simulink model "Ghost_f234"  (Simulink 8.1)
settings: Solver=ode1  StartTime=0.0  StopTime=inf  FixedStep=Ts  MaxStep=1e-3  RelTol=1e-3
PostLoadFcn:
  | NREL_Mode=1; BANSHEE_init;
InitFcn:
  | NREL_Mode=1; BANSHEE_init;
values from neighbouring files (symbols this model uses):
  DER_REL = xlsread('DER_relay.xlsx')    [relay_settings_init.m]
  F0 = xlsread('F0_relay_banshee.xlsx')    [relay_settings_init.m]
  F2 = xlsread('F2_relay_banshee.xlsx')    [relay_settings_init.m]
  F3 = xlsread('F3_relay_banshee.xlsx')    [relay_settings_init.m]
  F4 = xlsread('F4_relay_nrel.xlsx')    [relay_settings_init.m]
  Ts = 100E-6    (= 0.0001)    [BANSHEE_init.m]    (also in Ghost_init.m)
undefined symbols (not defined in the file or in its folder): CBID, communications_lib, Feeder2_lib, Feeder3_lib, Feeder4_lib, generic_ethernet_cb, Left, relay_housing_lib, SM_UtilityService, SS_COMMUNICATION, SS_F2_RELAY_HOUSING, SS_F3_RELAY_HOUSING, SS_Feeder2, SS_Feeder3, SS_Feeder4, Stim, type, utility_service_lib, V
libraries: simulink x80, relay_modbus_lib x80, breaker_lib x46, rtio_generic_modbus x45, cables_lib x30, rtlab x22, Load_lib x21, powerlib x20, transformer_lib x19, ssn_lib x13, artemis x6, BESS_lib x4
(part 1 of 6)
settings Model: ARTEMISmethode_block_infos=$$__separator__$$Ghost_f234/ARTEMIS Guide$$__separator__$$  Creator=RE25624  LastModifiedBy=hptb1  BufferReuse=off
settings SolverCC: ZeroCrossAlgorithm=Adaptive
settings DataIOCC: ExternalInput=getinputstruct(op_snapshot1)  InitialState=getstatestruct(op_snapshot1)  LimitDataPoints=off  MaxDataPoints=90060  SignalLoggingSaveFormat=Dataset  SaveOutput=off  SignalLogging=off  DSMLogging=off  SaveTime=off  OutputSaveName=result
settings OptimizationCC: BlockReduction=off  OptimizeBlockIOStorage=off  BufferReuse=off  ExpressionFolding=off  LocalBlockOutputs=off
settings DebuggingCC: MaxConsecutiveZCsMsg=warning  IgnoredZcDiagnostic=none  SolverPrmCheckMsg=none  MultiTaskRateTransMsg=warning  ParameterPrecisionLossMsg=none  FcnCallInpInsideContextMsg=EnableAllAsWarning  FrameProcessingCompatibilityMsg=error  ModelReferenceExtraNoncontSigs=warning  StrictBusMsg=Warning
settings ModelReferenceCC: UpdateModelReferenceTargets=IfOutOfDate
settings SFSimCC: SFSimEcho=off
settings GRTTargetCC: CodeReplacementLibrary=C89/C90 (ANSI)

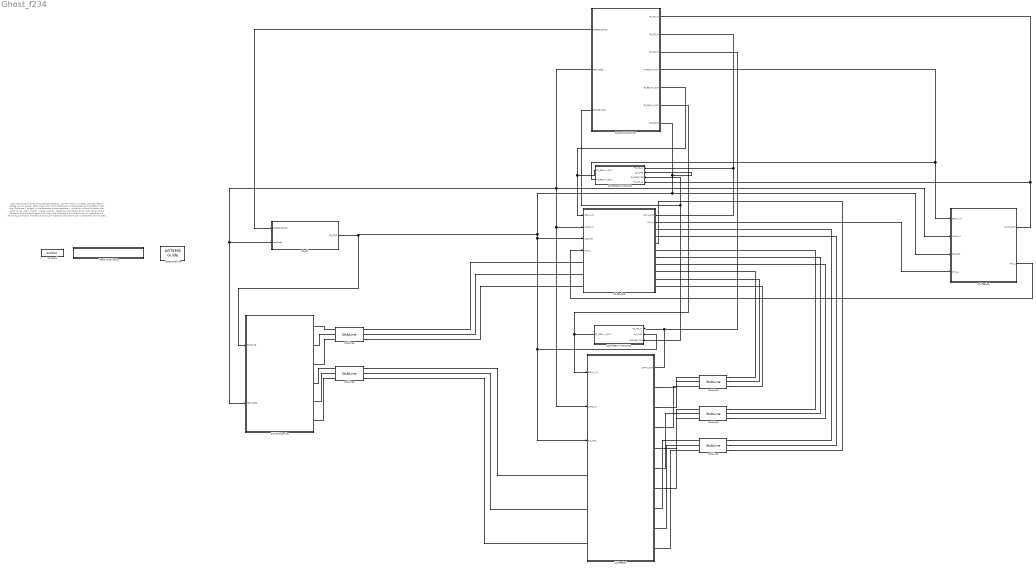
== system Ghost_f234 ==
  note: Copyright 2018 Alliance for Sustainable Energy, LLC
      |
      | Permission is hereby granted, free of charge, to any person obtaining a copy of this software
      | and associated documentation files (the "Software"), to deal in the Software without restriction,
      | including without limitation the rights to use, copy, modify, merge, publish, distribute, sublicense,
      | and/or sell copies of the Software, and to permit persons to whom the Software is furnished to do so,
      | subject to the following conditions:
      |
      | The above copyright notice and this permission notice shall be included in all copies or substantial portions of the Software.
      |
      | THE SOFTWARE IS PROVIDED "AS IS", WITHOUT WARRANTY OF ANY KIND, EXPRESS OR IMPLIED, INCLUDING
      | BUT NOT LIMITED TO THE WARRANTIES OF MERCHANTABILITY, FITNESS FOR A PARTICULAR PURPOSE AND
      | NONINFRINGEMENT. IN NO EVENT SHALL THE AUTHORS, THE COPYRIGHT HOLDERS, THE UNITED STATES,
      | THE UNITED STATES DEPARTMENT OF ENERGY, OR ANY OF THEIR EMPLOYEES BE LIABLE FOR ANY CLAIM,
      | DAMAGES OR OTHER LIABILITY, WHETHER IN AN ACTION OF CONTRACT, TORT OR OTHERWISE, ARISING FROM,
      | OUT OF OR IN CONNECTION WITH THE SOFTWARE OR THE USE OR OTHER DEALINGS IN THE SOFTWARE.
  ARTEMIS Guide : artemis/ARTEMIS/ARTEMIS Guide  Tag=FTSSmethode_opal_4hx0r99  Description=5.0_z1  lock=on  Ts=Ts  opt=art5  dyna=off  nb_perm=4  RT_fullcomp=off  ssn=on  ssn_itvc=off  ssn_ivic=off  ssn_ext=off  ssn_solver=Art5 with Backward Euler nodal interface  ssn_impulse=off  ssn_quasimpulse=off  ssn_impulse_loop=5  paraExtinctionThy=off  Thy_Impulse=on  dtc=Off  dtc_opt=normal  ao=on  simtype=off  ct_mac=off  lin_mov=off  lsp=[0.001 2]  spike_skip=Disabled  dtc_extra=1  dtc_sws=normal  dtc_pied=0.5  SPSRulesBlock=SPSRules  tre=on  ctmm=off  LF=off  dpl_type=ARTEMiS DPL  rlc_type=off  custom_type=off  para=on  ssn_ImpulseLoopBlockedStateUpdate=5  ssn_mov_iter_number=5  ssn_switch_iter_number=5  ssn_nib_type_verify=on
  Model Initialization : Subsystem  AncestorBlock=artemis/Tools /Misc/Model Initialization  mask(Model Functions){InitFcnX=NREL_Mode=1; BANSHEE_init;, prel=off, posl=on, inif=on, strf=off}
      mask prompts: InitFcnX "Initialisation"; prel "Preload Function"; posl "PostLoad Function"; inif "InitFcn"; strf "StartFcn"
      mask init:
      | currentBlock = gcb;
      | root = bdroot(currentBlock);
      | 
      | if ~strcmp(get_param(root,'BlockDiagramType'),'library')
      |     if prel==1
      |         set_param(root, 'PreLoadFcn', InitFcnX);
      |     else
      |         set_param(root, 'PreLoadFcn', '');
      |     end
      |     if inif==1
      |         set_param(root, 'InitFcn', InitFcnX);
      |     else
      |         set_param(root, 'InitFcn', '');
      |     end
      |     if strf==1
      |         set_param(root, 'StartFcn', InitFcnX);
      |     else
      |         set_param(root, 'StartFcn', '');
      |     end
      |     if posl==1
      |         set_param(root, 'PostLoadFcn', InitFcnX);
      |     else
      |         set_param(root, 'PostLoadFcn', '');
      |     end
      | end
      | 
      | pos = get_param(currentBlock, 'Position');
      | width = pos(3) - pos(1); height = pos(4) - pos(2);
      | txt = [ upper(root) '\n' '- InitFcn. . . . . '  get_param(root, 'InitFcn') ];
      settings: CopyFcn=set_param(gcb,'LinkStatus','inactive')
      mask Display: text(5, height*0.5, txt, 'horizontalAlignment', 'left', 'verticalAlignment', 'middle') ;
  SC_ctrl : Subsystem
  SM_UtilityService : Subsystem  AncestorBlock=utility_service_lib/SM_UtilityService
  SS_COMMUNICATION : Subsystem  AncestorBlock=communications_lib/SS_COMMUNICATION
  SS_F2_RELAY_HOUSING : Subsystem  AncestorBlock=relay_housing_lib/SS_F2_RELAY_HOUSING
  SS_F3_RELAY_HOUSING : Subsystem  AncestorBlock=relay_housing_lib/SS_F3_RELAY_HOUSING
  SS_Feeder2 : Subsystem  AncestorBlock=Feeder2_lib/SS_Feeder2
  SS_Feeder3 : Subsystem  AncestorBlock=Feeder3_lib/SS_Feeder3
  SS_Feeder4 : Subsystem  AncestorBlock=Feeder4_lib/SS_Feeder4
  StubLine1 : artemis/ARTEMIS/StubLine  Phases=3  pu=off  L=1500 * 9.43453e-08 / 2  Lpu=0.08  R=1500 * 2.28409e-5 / 2  Rpu=0.002  S_base=450e6/3  V_base=230e3/sqrt(3)  F_base=60  Ts=Ts
  StubLine2 : artemis/ARTEMIS/StubLine  Phases=3  pu=off  L=1500 * 9.43453e-08 / 2  Lpu=0.08  R=1500 * 2.28409e-5 / 2  Rpu=0.002  S_base=450e6/3  V_base=230e3/sqrt(3)  F_base=60  Ts=Ts
  StubLine3 : artemis/ARTEMIS/StubLine  Phases=3  pu=off  L=1500 * 9.43453e-08 / 2  Lpu=0.08  R=1500 * 2.28409e-5 / 2  Rpu=0.002  S_base=450e6/3  V_base=230e3/sqrt(3)  F_base=60  Ts=Ts
  StubLine8 : artemis/ARTEMIS/StubLine  Phases=3  pu=on  L=1500 * 9.43453e-08 / 2  Lpu=0.08  R=1500 * 2.28409e-5 / 2  Rpu=0.002  S_base=50e6/3  V_base=13.8e3/sqrt(3)  F_base=60  Ts=Ts
  StubLine9 : artemis/ARTEMIS/StubLine  Phases=3  pu=on  L=1500 * 9.43453e-08 / 2  Lpu=0.08  R=1500 * 2.28409e-5 / 2  Rpu=0.002  S_base=50e6/3  V_base=13.8e3/sqrt(3)  F_base=60  Ts=Ts
  powergui : powerlib/powergui  Priority=2  SimulationMode=Discrete  SolverType=Tustin  SampleTime=Ts  frequency=60  SPID=off  DisableSnubberDevices=off  DisableRonSwitches=off  DisableVfSwitches=off  SwTol=0  Interpol=off  DisplayEquations=off  frequencyindice=0  Pbase=100e6  ErrMax=1e-4  Iterations=50  UnitsV=kV  UnitsW=MW  FunctionMessages=off  echomessages=off  HookPort=off  EnableUseOfTLC=off  x0status=blocks  RestoreLinks=warning  ResistiveCurrentMeasurement=off  Frange=logspace(0,3,50)  Ylog=off  Xlog=off  ShowGrid=off  save=off  variable=ZData  structure=0  ZoomFFT=on  StartTime=0.0  cycles=2  DisplayStyle=off  fundamental=60  FreqAxis=off  MaxFrequency=1000  frequencyindicesteady=1  RmsSteady=1  display=off  Ts=0  methode=off
  wires:
  SS_Feeder3/1(DATA_OUT) -> SS_COMMUNICATION/2(F3_MS_IN), SS_F3_RELAY_HOUSING/1(F3_MS_IN)
  SS_F3_RELAY_HOUSING/1(F3_RELAY _OUT) -> SS_COMMUNICATION/5(F3_RELAY_OUT), SS_Feeder3/1(RELAY_IN)
  SS_F2_RELAY_HOUSING/1(F2_RELAY _OUT) -> SS_COMMUNICATION/6(F2_RELAY_OUT), SS_Feeder2/1(RELAY_IN)
  SS_Feeder2/1(DATA_OUT) -> SS_COMMUNICATION/3(F2_MS_IN), SS_F2_RELAY_HOUSING/1(F2_MS_IN)
  SS_COMMUNICATION/1(CMBNE_SGNLS) -> SC_ctrl/1(CMBNE_SGNLS)
  SC_ctrl/1(SC_CMD) -> SS_F2_RELAY_HOUSING/2(SC_CMD), SS_Feeder2/3(SC_CMD), SS_Feeder3/3(SC_CMD), SS_Feeder4/3(SC_CMD), SS_COMMUNICATION/7(CONSOLE), SS_F3_RELAY_HOUSING/2(SC_CMD), SM_UtilityService/1(CONSOLE)
  SS_F3_RELAY_HOUSING/2(F4_RELAY _OUT) -> SS_Feeder4/1(RELAY_IN), SS_COMMUNICATION/4(F4_RELAY_OUT)
  SS_Feeder4/1(DATA_OUT) -> SS_COMMUNICATION/1(F4_MS_IN), SS_F3_RELAY_HOUSING/4(F4_MS_IN)
  SS_Feeder3/2(PHIL_V) -> SS_Feeder4/4(PHIL_V)
  SS_Feeder4/2(PHIL_I) -> SS_Feeder3/4(PHIL_I)
  SS_COMMUNICATION/3(GOOSE_TRIP) -> SS_F3_RELAY_HOUSING/3(GOOSE_TRIP), SS_F2_RELAY_HOUSING/3(GOOSE_TRIP)
  SS_COMMUNICATION/2(TEST_SEQ) -> SS_Feeder2/2(LOAD_IN), SS_Feeder3/2(LOAD_IN), SM_UtilityService/2(TEST_SEQ), SC_ctrl/2(TestData), SS_Feeder4/2(LOAD_IN)
  connections:
  SS_Feeder2/RConn2 -- StubLine1/LConn2
  SS_Feeder2/RConn1 -- StubLine1/LConn1
  SS_Feeder2/RConn3 -- StubLine1/LConn3
  StubLine2/LConn2 -- SS_Feeder2/RConn5
  StubLine2/LConn3 -- SS_Feeder2/RConn6
  StubLine2/LConn1 -- SS_Feeder2/RConn4
  StubLine3/LConn2 -- SS_Feeder2/RConn8
  StubLine3/LConn1 -- SS_Feeder2/RConn7
  StubLine3/LConn3 -- SS_Feeder2/RConn9
  StubLine3/RConn3 -- SS_Feeder3/RConn3
  StubLine3/RConn2 -- SS_Feeder3/RConn2
  StubLine3/RConn1 -- SS_Feeder3/RConn1
  StubLine2/RConn3 -- SS_Feeder3/RConn6
  StubLine2/RConn1 -- SS_Feeder3/RConn4
  StubLine1/RConn3 -- SS_Feeder3/RConn9
  StubLine1/RConn2 -- SS_Feeder3/RConn8
  StubLine1/RConn1 -- SS_Feeder3/RConn7
  StubLine8/LConn1 -- SM_UtilityService/RConn1
  StubLine8/LConn2 -- SM_UtilityService/RConn2
  StubLine8/LConn3 -- SM_UtilityService/RConn3
  StubLine9/LConn2 -- SM_UtilityService/RConn5
  StubLine9/LConn3 -- SM_UtilityService/RConn6
  StubLine9/LConn1 -- SM_UtilityService/RConn4
  StubLine8/RConn3 -- SS_Feeder3/LConn3
  StubLine8/RConn2 -- SS_Feeder3/LConn2
  StubLine8/RConn1 -- SS_Feeder3/LConn1
  StubLine9/RConn1 -- SS_Feeder2/LConn1
  StubLine9/RConn2 -- SS_Feeder2/LConn2
  StubLine9/RConn3 -- SS_Feeder2/LConn3
  SS_Feeder3/RConn5 -- StubLine2/RConn2

== system Ghost_f234/Model Initialization ==

== system Ghost_f234/SC_ctrl ==
  note: % Copyright (c) 2016 Massachusetts Institute of Technology
      | % Permission is hereby granted, free of charge, to any person obtaining a copy of this
      | % software and associated documentation files (the "Software"), to deal in the Software
      | % without restriction, including without limitation the rights to use, copy, modify,
      | % merge, publish, distribute, sublicense, and/or sell copies of the Software, and to
      | % permit persons to whom the Software is furnished to do so, subject to the following
      | % conditions:
      | %
      | %
      | % The above copyright notice and this permission notice shall be included in
      | % all copies or substantial portions of the Software.
      | %
      | % THE SOFTWARE IS PROVIDED "AS IS", WITHOUT WARRANTY OF ANY KIND, EXPRESS OR IMPLIED,
      | % INCLUDING BUT NOT LIMITED TO THE WARRANTIES OF MERCHANTABILITY, FITNESS FOR A
      | % PARTICULAR PURPOSE AND NONINFRINGEMENT. IN NO EVENT SHALL THE AUTHORS OR COPYRIGHT
      | % HOLDERS BE LIABLE FOR ANY CLAIM, DAMAGES OR OTHER LIABILITY, WHETHER IN AN ACTION
      | % OF CONTRACT, TORT OR OTHERWISE, ARISING FROM, OUT OF OR IN CONNECTION WITH THE
      | % SOFTWARE OR THE USE OR OTHER DEALINGS IN THE SOFTWARE.
      | %
      | %
      | %%
  CMBNE_SGNLS : Inport
  TestData : Inport  Port=2
  Bus Creator1 : BusCreator  Inputs=11
  Bus Creator2 : BusCreator  Inputs=2
  Bus Selector : BusSelector  OutputSignals=F2_MS_IN
  Bus Selector{6..7,10,12,14} (5 alike) : BusSelector  OutputSignals=Status
  Bus Selector11 : BusSelector  OutputSignals=F3_MS_IN.CB_DATA.F3_PCC,F3_MS_IN.CB_DATA.F3_CB_10
  Bus Selector13 : BusSelector  OutputSignals=ESS_DATA
  Bus Selector15 : BusSelector  OutputSignals=Battery.SoC
  Bus Selector16 : BusSelector  OutputSignals=F4_MS_IN
  Bus Selector17 : BusSelector  OutputSignals=ESS_DATA
  Bus Selector18 : BusSelector  OutputSignals=Battery.SoC
  Bus Selector5 : BusSelector  OutputSignals=F3_MS_IN.CB_DATA.F3_PCC,F3_MS_IN.CB_DATA.F3_CB_3,F3_MS_IN.NG_CHP_DATA
  Bus Selector8 : BusSelector  OutputSignals=cb.cb_meas
  CB_modbus_mock : Subsystem
  DO NOT WRITE : Constant  Value=0
  Gen1_Modbus_Stimuli2 : Subsystem
  Gen2_NGCHP_Modbus_Stimuli : Subsystem
  Gen3_Modbus_Stimuli1 : Subsystem
  IO_scaling : Subsystem
  Logical Operator1 : Logic  Inputs=3  AllPortsSameDT=off  OutDataTypeStr=boolean
  Logical Operator2 : Logic  Inputs=3  AllPortsSameDT=off  OutDataTypeStr=boolean
  Manual Switch : ManualSwitch
  Manual Switch1 : ManualSwitch
  OpComm : rtlab/OpComm  nbport=2  groupe_acq=1  subsys_rate=0  st=0  Synchronization=on  Interpolation=on  Threshold=1.0  Missed_Data=off  Sim_Time=off  Samples=off  dynSigOut=off  from_console=0  warning_done=off  writeOpCommFile=off  Offset=off
  PV1 control : Subsystem
  PV2 control : Subsystem
  Plots : Subsystem
  SOC1 control : Subsystem
  SOC2 control : Subsystem
  TestSeq : Subsystem
  TestSequenceGen : Subsystem
  WRITE : Constant
  SC_CMD : Outport
  wires:
  CMBNE_SGNLS/1 -> OpComm/1
  Bus Creator1/1 -> SC_CMD/1
  Manual Switch/1 -> Bus Creator2/1  "record_rms_signals"
  Manual Switch1/1 -> Bus Creator2/2  "record_inst_signals"
  Bus Creator2/1 -> [data_logging]  "DataLogging"
  TestData/1 -> OpComm/2
  WRITE/1 -> Manual Switch1/2, Manual Switch/2  "record_rms_signals"
  DO NOT WRITE/1 -> Manual Switch1/1, Manual Switch/1
  [data_logging] -> Bus Creator1/4  "DataLogging"
  CB_modbus_mock/1(Out1) -> Bus Creator1/7  "CBStimuli"
  Gen1_Modbus_Stimuli2/1(MbCtrl) -> Bus Creator1/8  "Gen1"
  SOC2 control/1(Out1) -> Bus Creator1/5  "ESS2_ctrl"
  PV2 control/1(Out1) -> Bus Creator1/6  "PV2_ctrl"
  OpComm/1 -> [CMBNE], Bus Selector11/1, Bus Selector5/1, Plots/1(CMBNE_SGNLS)
  Gen2_NGCHP_Modbus_Stimuli/1(MbCtrl) -> Bus Creator1/9  "CHP_cmds"
  Bus Selector5/1 -> Bus Selector6/1  "<F3_PCC>"
  Bus Selector5/3 -> Bus Selector8/1  "<NG_CHP_DATA>"
  Bus Selector6/1 -> Logical Operator1/1  "<Status>"
  Bus Selector7/1 -> Logical Operator1/3  "<Status>"
  Bus Selector8/1 -> Bus Selector7/1  "<cb_meas>"
  Logical Operator1/1 -> Gen2_NGCHP_Modbus_Stimuli/1(MainsCon)
  Bus Selector10/1 -> Logical Operator1/2  "<Status>"
  Bus Selector5/2 -> Bus Selector10/1  "<F3_CB_3>"
  Gen3_Modbus_Stimuli1/1(MbCtrl) -> Bus Creator1/10  "Gen3_ctrl"
  Logical Operator2/1 -> Gen3_Modbus_Stimuli1/1(MainsCon)
  Bus Selector11/1 -> Bus Selector12/1  "<F3_PCC>"
  Bus Selector12/1 -> Logical Operator2/1  "<Status>"
  Bus Selector11/2 -> Bus Selector14/1  "<F3_CB_10>"
  Bus Selector14/1 -> Logical Operator2/3, Logical Operator2/2  "<Status>"
  OpComm/2 -> TestSeq/1(TestData)
  IO_scaling/1(Out1) -> Bus Creator1/11  "IO_scaling"
  TestSequenceGen/1(Out1) -> Bus Creator1/1  "TestSeq"
  SOC1 control/1(Out1) -> Bus Creator1/2  "ESS1_ctrl"
  PV1 control/1(Out1) -> Bus Creator1/3  "PV1_ctrl"
  [CMBNE] -> Bus Selector/1
  Bus Selector/1 -> Bus Selector13/1  "<F2_MS_IN>"
  Bus Selector13/1 -> Bus Selector15/1  "<ESS_DATA>"
  Bus Selector15/1 -> SOC1 control/1(SOC)  "<SoC>"
  [CMBNE] -> Bus Selector16/1
  Bus Selector16/1 -> Bus Selector17/1  "<F4_MS_IN>"
  Bus Selector17/1 -> Bus Selector18/1  "<ESS_DATA>"
  Bus Selector18/1 -> SOC2 control/1(SOC)  "<SoC>"

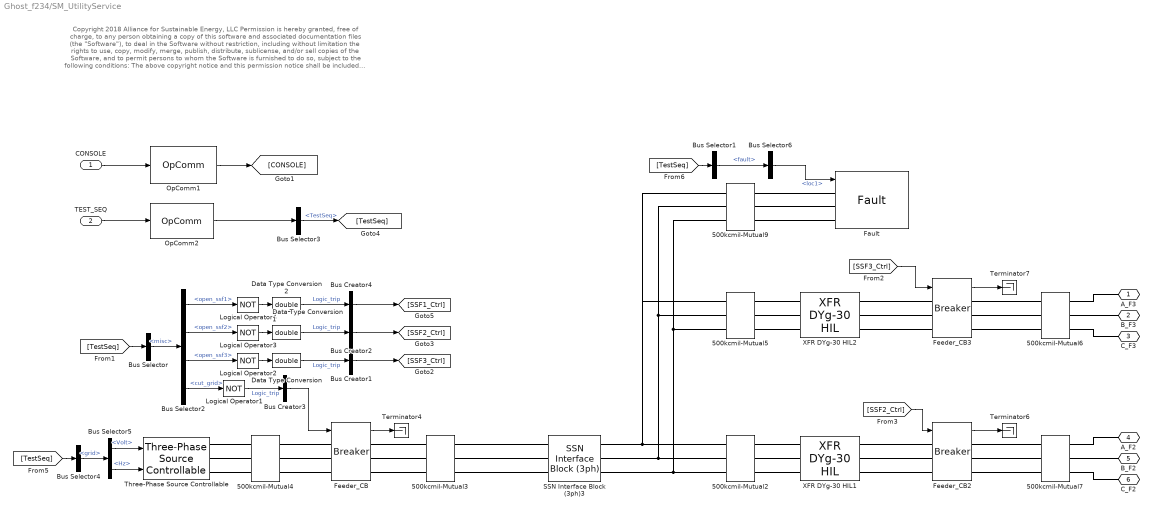
== system Ghost_f234/SM_UtilityService ==
  note: Copyright 2018 Alliance for Sustainable Energy, LLC
      |
      | Permission is hereby granted, free of charge, to any person obtaining a copy of this software
      | and associated documentation files (the "Software"), to deal in the Software without restriction,
      | including without limitation the rights to use, copy, modify, merge, publish, distribute, sublicense,
      | and/or sell copies of the Software, and to permit persons to whom the Software is furnished to do so,
      | subject to the following conditions:
      |
      | The above copyright notice and this permission notice shall be included in all copies or substantial portions of the Software.
      |
      | THE SOFTWARE IS PROVIDED "AS IS", WITHOUT WARRANTY OF ANY KIND, EXPRESS OR IMPLIED, INCLUDING
      | BUT NOT LIMITED TO THE WARRANTIES OF MERCHANTABILITY, FITNESS FOR A PARTICULAR PURPOSE AND
      | NONINFRINGEMENT. IN NO EVENT SHALL THE AUTHORS, THE COPYRIGHT HOLDERS, THE UNITED STATES,
      | THE UNITED STATES DEPARTMENT OF ENERGY, OR ANY OF THEIR EMPLOYEES BE LIABLE FOR ANY CLAIM,
      | DAMAGES OR OTHER LIABILITY, WHETHER IN AN ACTION OF CONTRACT, TORT OR OTHERWISE, ARISING FROM,
      | OUT OF OR IN CONNECTION WITH THE SOFTWARE OR THE USE OR OTHER DEALINGS IN THE SOFTWARE.
  CONSOLE : Inport
  TEST_SEQ : Inport  Port=2
  500kcmil-Mutual2 : cables_lib/500kcmil-Mutual  length=200  par_sets=1  ratio=3
  500kcmil-Mutual{3..4,6..7} (4 alike) : cables_lib/500kcmil-Mutual  length=50  par_sets=1  ratio=3
  500kcmil-Mutual5 : cables_lib/500kcmil-Mutual  length=200  par_sets=1  ratio=3
  500kcmil-Mutual9 : cables_lib/500kcmil-Mutual  length=200  par_sets=1  ratio=3
  Bus Creator{1..4} (4 alike) : BusCreator  Inputs=1
  Bus Selector : BusSelector  OutputSignals=misc
  Bus Selector1 : BusSelector  OutputSignals=fault
  Bus Selector2 : BusSelector  OutputSignals=open_ssf1,open_ssf2,open_ssf3,cut_grid
  Bus Selector3 : BusSelector  OutputSignals=TestSeq
  Bus Selector4 : BusSelector  OutputSignals=grid
  Bus Selector5 : BusSelector  OutputSignals=Volt,Hz
  Bus Selector6 : BusSelector  OutputSignals=loc1
  Data Type Conversion : DataTypeConversion  OutDataTypeStr=double
  Data Type Conversion1 : DataTypeConversion  OutDataTypeStr=double
  Data Type Conversion2 : DataTypeConversion  OutDataTypeStr=double
  Fault : fault_lib/Fault  FaultResistance=0.1  GroundResistance=1.73  SnubberResistance=1E6
  Feeder_CB : breaker_lib/Breaker  Ts=Ts  mech_delay=cb_mech_delay
  Feeder_CB2 : breaker_lib/Breaker  Ts=Ts  mech_delay=cb_mech_delay
  Feeder_CB3 : breaker_lib/Breaker  Ts=Ts  mech_delay=cb_mech_delay
  Logical Operator{1..4} (4 alike) : Logic  Operator=NOT  AllPortsSameDT=off  OutDataTypeStr=boolean
  OpComm1 : rtlab/OpComm  nbport=1  groupe_acq=1  subsys_rate=0  st=0  Synchronization=on  Interpolation=on  Threshold=1.0  Missed_Data=off  Sim_Time=off  Samples=off  dynSigOut=off  from_console=1  warning_done=off  writeOpCommFile=off  Offset=off
  OpComm2 : rtlab/OpComm  nbport=1  groupe_acq=1  subsys_rate=0  st=0  Synchronization=on  Interpolation=on  Threshold=1.0  Missed_Data=off  Sim_Time=off  Samples=off  dynSigOut=off  from_console=0  warning_done=off  writeOpCommFile=off  Offset=off
  SSN Interface Block (3ph)3 : ssn_lib/SSN Interface Block (3ph)  nb_phase=3  nb_port=2  p1_type=V-type(Left)  p2_type=V-type (Right)  p3_type=V-type(Left)  p4_type=V-type(Left)  p5_type=V-type(Left)  p6_type=V-type(Left)  p7_type=V-type(Left)  p8_type=V-type(Left)  p9_type=V-type(Left)  p10_type=V-type(Left)  p11_type=V-type(Left)  p12_type=V-type(Left)  p13_type=V-type(Left)  p14_type=V-type(Left)  p15_type=V-type(Left)  p16_type=V-type(Left)  I_port_shunt_resistance=1e9
  Terminator4 : Terminator
  Terminator6 : Terminator
  Terminator7 : Terminator
  Three-Phase Source Controllable : controllable_grid_lib/Three-Phase Source Controllable  Ts=Ts  Rg=0.8  Lg=16.58e-3  mask{Ts=Ts}
  XFR DYg-30 HIL1 : transformer_lib/XFR DYg-30 HIL  Rating=50000  Vp=115000  Vs=13800  Z=6  XR=30
  XFR DYg-30 HIL2 : transformer_lib/XFR DYg-30 HIL  Rating=50000  Vp=115000  Vs=13800  Z=6  XR=30
  A_F3 : PMIOPort  Port=1  Side=Right
  B_F3 : PMIOPort  Port=2  Side=Right
  C_F3 : PMIOPort  Port=3  Side=Right
  A_F2 : PMIOPort  Port=4  Side=Right
  B_F2 : PMIOPort  Port=5  Side=Right
  C_F2 : PMIOPort  Port=6  Side=Right
  wires:
  CONSOLE/1 -> OpComm1/1
  OpComm1/1 -> [CONSOLE]
  Feeder_CB/1 -> Terminator4/1
  Feeder_CB2/1 -> Terminator6/1
  Feeder_CB3/1 -> Terminator7/1
  TEST_SEQ/1 -> OpComm2/1
  [TestSeq] -> Bus Selector/1
  Logical Operator1/1 -> Bus Creator3/1  "Logic_trip"
  Bus Creator3/1 -> Feeder_CB/1
  Bus Selector/1 -> Bus Selector2/1  "<misc>"
  Bus Selector2/4 -> Logical Operator1/1  "<cut_grid>"
  Bus Selector2/3 -> Logical Operator2/1  "<open_ssf3>"
  Logical Operator2/1 -> Data Type Conversion/1
  Bus Creator1/1 -> [SSF3_Ctrl]
  Data Type Conversion/1 -> Bus Creator1/1  "Logic_trip"
  Bus Selector3/1 -> [TestSeq]  "<TestSeq>"
  OpComm2/1 -> Bus Selector3/1
  Bus Selector2/2 -> Logical Operator3/1  "<open_ssf2>"
  Logical Operator3/1 -> Data Type Conversion1/1
  Bus Creator2/1 -> [SSF2_Ctrl]
  Data Type Conversion1/1 -> Bus Creator2/1  "Logic_trip"
  Bus Selector2/1 -> Logical Operator4/1  "<open_ssf1>"
  Logical Operator4/1 -> Data Type Conversion2/1
  Bus Creator4/1 -> [SSF1_Ctrl]
  Data Type Conversion2/1 -> Bus Creator4/1  "Logic_trip"
  [SSF3_Ctrl] -> Feeder_CB3/1
  [SSF2_Ctrl] -> Feeder_CB2/1
  [TestSeq] -> Bus Selector4/1
  Bus Selector4/1 -> Bus Selector5/1  "<grid>"
  Bus Selector5/2 -> Three-Phase Source Controllable/2  "<Hz>"
  Bus Selector5/1 -> Three-Phase Source Controllable/1  "<Volt>"
  [TestSeq] -> Bus Selector1/1
  Bus Selector1/1 -> Bus Selector6/1  "<fault>"
  Bus Selector6/1 -> Fault/1  "<loc1>"
  connections:
  500kcmil-Mutual3/LConn3 -- Feeder_CB/RConn3
  500kcmil-Mutual3/LConn1 -- Feeder_CB/RConn1
  500kcmil-Mutual3/LConn2 -- Feeder_CB/RConn2
  SSN Interface Block (3ph)3/LConn2 -- 500kcmil-Mutual3/RConn2
  SSN Interface Block (3ph)3/LConn1 -- 500kcmil-Mutual3/RConn1
  SSN Interface Block (3ph)3/LConn3 -- 500kcmil-Mutual3/RConn3
  500kcmil-Mutual4/RConn3 -- Feeder_CB/LConn3
  500kcmil-Mutual4/RConn2 -- Feeder_CB/LConn2
  500kcmil-Mutual4/RConn1 -- Feeder_CB/LConn1
  Three-Phase Source Controllable/RConn3 -- 500kcmil-Mutual4/LConn3
  Three-Phase Source Controllable/RConn1 -- 500kcmil-Mutual4/LConn1
  Three-Phase Source Controllable/RConn2 -- 500kcmil-Mutual4/LConn2
  500kcmil-Mutual2/RConn2 -- XFR DYg-30 HIL1/LConn2
  500kcmil-Mutual2/RConn1 -- XFR DYg-30 HIL1/LConn1
  500kcmil-Mutual2/RConn3 -- XFR DYg-30 HIL1/LConn3
  500kcmil-Mutual5/RConn2 -- XFR DYg-30 HIL2/LConn2
  500kcmil-Mutual5/RConn1 -- XFR DYg-30 HIL2/LConn1
  500kcmil-Mutual5/RConn3 -- XFR DYg-30 HIL2/LConn3
  SSN Interface Block (3ph)3/RConn1 -- 500kcmil-Mutual2/LConn1 -- 500kcmil-Mutual5/LConn1 -- 500kcmil-Mutual9/LConn1
  500kcmil-Mutual5/LConn2 -- SSN Interface Block (3ph)3/RConn2 -- 500kcmil-Mutual2/LConn2 -- 500kcmil-Mutual9/LConn2
  500kcmil-Mutual5/LConn3 -- SSN Interface Block (3ph)3/RConn3 -- 500kcmil-Mutual2/LConn3 -- 500kcmil-Mutual9/LConn3
  XFR DYg-30 HIL2/RConn1 -- Feeder_CB3/LConn1
  XFR DYg-30 HIL2/RConn2 -- Feeder_CB3/LConn2
  XFR DYg-30 HIL2/RConn3 -- Feeder_CB3/LConn3
  XFR DYg-30 HIL1/RConn3 -- Feeder_CB2/LConn3
  XFR DYg-30 HIL1/RConn2 -- Feeder_CB2/LConn2
  XFR DYg-30 HIL1/RConn1 -- Feeder_CB2/LConn1
  500kcmil-Mutual6/LConn2 -- Feeder_CB3/RConn2
  500kcmil-Mutual6/LConn3 -- Feeder_CB3/RConn3
  500kcmil-Mutual6/LConn1 -- Feeder_CB3/RConn1
  500kcmil-Mutual7/LConn2 -- Feeder_CB2/RConn2
  500kcmil-Mutual7/LConn3 -- Feeder_CB2/RConn3
  500kcmil-Mutual7/LConn1 -- Feeder_CB2/RConn1
  B_F2/RConn1 -- 500kcmil-Mutual7/RConn2
  A_F2/RConn1 -- 500kcmil-Mutual7/RConn1
  C_F2/RConn1 -- 500kcmil-Mutual7/RConn3
  B_F3/RConn1 -- 500kcmil-Mutual6/RConn2
  A_F3/RConn1 -- 500kcmil-Mutual6/RConn1
  C_F3/RConn1 -- 500kcmil-Mutual6/RConn3
  500kcmil-Mutual9/RConn2 -- Fault/LConn2
  500kcmil-Mutual9/RConn3 -- Fault/LConn3
  500kcmil-Mutual9/RConn1 -- Fault/LConn1

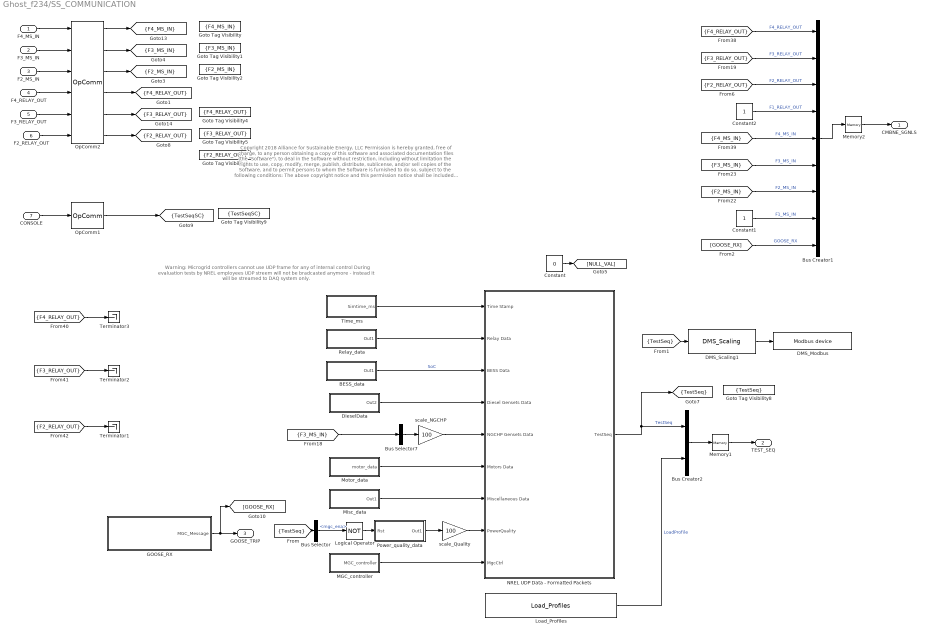
== system Ghost_f234/SS_COMMUNICATION ==
  note: Warning: Microgrid controllers cannot use UDP frame for any of internal control
      | During evaluation tests by NREL employees UDP streem will not be bradcasted anymore - instead it will
      | be streamed to DAQ system only.
  note: Copyright 2018 Alliance for Sustainable Energy, LLC
      |
      | Permission is hereby granted, free of charge, to any person obtaining a copy of this software
      | and associated documentation files (the "Software"), to deal in the Software without restriction,
      | including without limitation the rights to use, copy, modify, merge, publish, distribute, sublicense,
      | and/or sell copies of the Software, and to permit persons to whom the Software is furnished to do so,
      | subject to the following conditions:
      |
      | The above copyright notice and this permission notice shall be included in all copies or substantial portions of the Software.
      |
      | THE SOFTWARE IS PROVIDED "AS IS", WITHOUT WARRANTY OF ANY KIND, EXPRESS OR IMPLIED, INCLUDING
      | BUT NOT LIMITED TO THE WARRANTIES OF MERCHANTABILITY, FITNESS FOR A PARTICULAR PURPOSE AND
      | NONINFRINGEMENT. IN NO EVENT SHALL THE AUTHORS, THE COPYRIGHT HOLDERS, THE UNITED STATES,
      | THE UNITED STATES DEPARTMENT OF ENERGY, OR ANY OF THEIR EMPLOYEES BE LIABLE FOR ANY CLAIM,
      | DAMAGES OR OTHER LIABILITY, WHETHER IN AN ACTION OF CONTRACT, TORT OR OTHERWISE, ARISING FROM,
      | OUT OF OR IN CONNECTION WITH THE SOFTWARE OR THE USE OR OTHER DEALINGS IN THE SOFTWARE.
  F4_MS_IN : Inport
  F3_MS_IN : Inport  Port=2
  F2_MS_IN : Inport  Port=3
  F4_RELAY_OUT : Inport  Port=4
  F3_RELAY_OUT : Inport  Port=5
  F2_RELAY_OUT : Inport  Port=6
  CONSOLE : Inport  Port=7
  BESS_data : Subsystem
  Bus Creator1 : BusCreator  Inputs=9
  Bus Creator2 : BusCreator  Inputs=2
  Bus Selector : BusSelector  OutputSignals=misc.mgc_ena
  Bus Selector7 : BusSelector  OutputSignals=NG_CHP_DATA.cb.relay_out.m.Vpu,NG_CHP_DATA.CHPData.TempActual,NG_CHP_DATA.CHPData.Thermal data.Heat_Recovered_MBtu_hr,NG_CHP_DATA.CHPData.Thermal data.Nm3_per_hour_NG_fuel_usage,NG_CHP_DATA.CHPData.Thermal data.CO2_lbm_hr,NG_CHP_DATA.CHPData.HeatFromBoiler MBtu/hr,NG_CHP_DATA.CHPData.CHPHeatContribution MBtu/hr,NG_CHP_DATA.CHPData.Boiler_Nm^3/hr ,NG_CHP_DATA.CHPData.Boiler lbm/hr CO2  OutputAsBus=on
  Constant : Constant  Value=0
  Constant1 : Constant
  Constant2 : Constant
  DMS_Modbus : rtio_generic_modbus/Modbus device  conf_name=DMS_cfg.opal  conf_name_mask=DMS_cfg.xls  sample_time=Ts
  DMS_Scaling1 : DMS_slave_lib/DMS_Scaling
  DieselData : Subsystem
  "GOOSE_RX " : Subsystem
  Goto Tag Visibility : GotoTagVisibility  GotoTag=F4_MS_IN
  Goto Tag Visibility1 : GotoTagVisibility  GotoTag=F3_MS_IN
  Goto Tag Visibility2 : GotoTagVisibility  GotoTag=F2_MS_IN
  Goto Tag Visibility4 : GotoTagVisibility  GotoTag=F4_RELAY_OUT
  Goto Tag Visibility5 : GotoTagVisibility  GotoTag=F3_RELAY_OUT
  Goto Tag Visibility6 : GotoTagVisibility  GotoTag=F2_RELAY_OUT
  Goto Tag Visibility8 : GotoTagVisibility  GotoTag=TestSeq
  Goto Tag Visibility9 : GotoTagVisibility  GotoTag=TestSeqSC
  Load_Profiles : LoadProfiles_lib/Load_Profiles
  Logical Operator : Logic  Operator=NOT  AllPortsSameDT=off  OutDataTypeStr=boolean
  MGC_controller : Subsystem
  Memory1 : Memory
  Memory2 : Memory
  Misc_data : Subsystem
  Motor_data : Subsystem
  NREL UDP Data - Formatted Packets : Subsystem  AncestorBlock=NREL_UDP_lib/NREL UDP Data - Formatted Packets  mask(UDP Data Block){ProfileID=6, NumOfRelays=[59, [1, 1, 1000, 100]], NumOfBatteries=2, NumOfDieselGensets=[2, [100, 100]], NumOfNGCHPGensets=[1, [100, 100, 100, 100, 100, 100, 100, 100, 100]], NumOfMotors=2, NumOfQuality=[23 10 10], NumOfMiscellaneousDataScales=2, NumOfMiscellaneousDataSignalsScales=[[50, 1], [8, 1]]}
      mask prompts: ProfileID "Profile ID"; NumOfRelays "Relay Data"; NumOfBatteries "# of Batteries"; NumOfDieselGensets "Diesel Gensets Data"; NumOfNGCHPGensets "NG-CHP Gensets Data"; NumOfMotors "# of Motors"; NumOfQuality "Power quality"; NumOfMiscellaneousDataScales "Misc. Data - No. of Scale Factors"; NumOfMiscellaneousDataSignalsScales "Misc. - No. Signals and Scale Values"
      mask help:
      | * All signal scaling/modifications should be external to this block
      |
      | Profile ID: (1-Sheriff, 2-Banshee, 3-Canary, 4-Siren, 5-NREL)
      |
      | Relay Data: No. of relays feeding packet data to breakers in display - mapped/indexed in ascending order
      | -Packet order: Active power(kW), reactive power(kVAR), voltage(per-unit), frequency (Hz), breaker status (1:closed, 0:open)
      | -Input format: [No. of Relays, [scale_kW, scale_kVAR, scale_Vpu, scale_Hz]]
      | -Ex:[4, [10, 10, 100, 100]]
      |
      | No. of Batteries: TBD
      | -Ex: [0]
      |
      | No. of Diesel Gensets: No. of diesel gensets in the system feeding data to the display.
      | -Packet order: terminal voltage(per-unit), fuel consumption (Gals/hr)
      | -Input format: [No. of gensets, [scale_Vpu, scale_fuel]]
      | -Ex: [0, [1,1]]
      |
      | No. of NG/CHP Gensets: No. of NGCHP gensets in the system feeding data to the display.
      | -Packet order: Terminal Vpu, Temp Actual, Heat Recovered, Fuel usage, CHP CO2, Heat from boiler, CHP heat contribution, Boiler Nm^3/hr, Boiler lbm/hr CO2
      | -Ex: [1, [100,100,100,100,100,100,100,100,100]]
      |
      | Motors Data: No. of motors monitored in the system. Currently, only looking at motor on/off state.
      | -Input format: [No. of motors]
      | -Ex: [1]
      |
      | Misc. Data - No. of Scale factor: No. of scale factors to be applied to each signal-set.
      | -Ex: [3]
      |
      | Misc. Data - No. of Signals and Scale Values: Size of signal set and scale value to be applied to the signal-set.
      | -Ex: [[1, 1000], [6, 100], [3, 10]]
  OpComm1 : rtlab/OpComm  nbport=1  groupe_acq=1  subsys_rate=0  st=0  Synchronization=on  Interpolation=on  Threshold=1.0  Missed_Data=off  Sim_Time=off  Samples=off  dynSigOut=off  from_console=1  warning_done=off  writeOpCommFile=off  Offset=off
  OpComm2 : rtlab/OpComm  nbport=6  groupe_acq=1  subsys_rate=0  st=0  Synchronization=on  Interpolation=on  Threshold=1.0  Missed_Data=off  Sim_Time=off  Samples=off  dynSigOut=off  from_console=0  warning_done=off  writeOpCommFile=off  Offset=off
  Power_quality_data : Subsystem
  Relay_data : Subsystem
  Terminator1 : Terminator
  Terminator2 : Terminator
  Terminator3 : Terminator
  Time_ms : Subsystem
  scale_NGCHP : Gain  Gain=100
  scale_Quality : Gain  Gain=100
  CMBNE_SGNLS : Outport
  TEST_SEQ : Outport  Port=2
  GOOSE_TRIP : Outport  Port=3
  tag scope: F2_MS_IN=scoped, F2_RELAY_OUT=scoped, F3_MS_IN=scoped, F3_RELAY_OUT=scoped, F4_MS_IN=scoped, F4_RELAY_OUT=scoped, TestSeq=scoped, TestSeqSC=scoped
  wires:
  Load_Profiles/1 -> Bus Creator2/2  "LoadProfile"
  F3_MS_IN/1 -> OpComm2/2
  Memory1/1 -> TEST_SEQ/1
  F2_RELAY_OUT/1 -> OpComm2/6
  F2_MS_IN/1 -> OpComm2/3
  Constant/1 -> [NULL_VAL]
  [F3_MS_IN] -> Bus Selector7/1
  Bus Selector7/1 -> scale_NGCHP/1
  scale_NGCHP/1 -> NREL UDP Data - Formatted Packets/5(NGCHP Gensets Data)
  Memory2/1 -> CMBNE_SGNLS/1
  Bus Creator1/1 -> Memory2/1
  Constant1/1 -> Bus Creator1/8  "F1_MS_IN"
  [F2_RELAY_OUT] -> Bus Creator1/3  "F2_RELAY_OUT"
  Constant2/1 -> Bus Creator1/4  "F1_RELAY_OUT"
  [F3_RELAY_OUT] -> Bus Creator1/2  "F3_RELAY_OUT"
  [F3_MS_IN] -> Bus Creator1/6  "F3_MS_IN"
  [F2_MS_IN] -> Bus Creator1/7  "F2_MS_IN"
  Time_ms/1(Simtime_ms) -> NREL UDP Data - Formatted Packets/1(Time Stamp)
  F4_MS_IN/1 -> OpComm2/1
  F4_RELAY_OUT/1 -> OpComm2/4
  F3_RELAY_OUT/1 -> OpComm2/5
  OpComm2/1 -> [F4_MS_IN]
  OpComm2/2 -> [F3_MS_IN]
  OpComm2/3 -> [F2_MS_IN]
  OpComm2/4 -> [F4_RELAY_OUT]
  OpComm2/5 -> [F3_RELAY_OUT]
  OpComm2/6 -> [F2_RELAY_OUT]
  [F4_RELAY_OUT] -> Bus Creator1/1  "F4_RELAY_OUT"
  [F4_MS_IN] -> Bus Creator1/5  "F4_MS_IN"
  [F4_RELAY_OUT] -> Terminator3/1
  [F3_RELAY_OUT] -> Terminator2/1
  [F2_RELAY_OUT] -> Terminator1/1
  "GOOSE_RX "/1(MGC_Message) -> [GOOSE_RX], GOOSE_TRIP/1
  Relay_data/1(Out1) -> NREL UDP Data - Formatted Packets/2(Relay Data)
  Misc_data/1(Out1) -> NREL UDP Data - Formatted Packets/7(Miscellaneous Data)
  Motor_data/1(motor_data) -> NREL UDP Data - Formatted Packets/6(Motors Data)
  NREL UDP Data - Formatted Packets/1(TestSeq) -> [TestSeq], Bus Creator2/1  "TestSeq"
  Bus Creator2/1 -> Memory1/1
  CONSOLE/1 -> OpComm1/1
  OpComm1/1 -> [TestSeqSC]
  BESS_data/1(Out1) -> NREL UDP Data - Formatted Packets/3(BESS Data)  "SoC"
  DieselData/1(Out2) -> NREL UDP Data - Formatted Packets/4(Diesel Gensets Data)
  Power_quality_data/1(Out1) -> scale_Quality/1
  [TestSeq] -> Bus Selector/1
  Bus Selector/1 -> Logical Operator/1  "<mgc_ena>"
  Logical Operator/1 -> Power_quality_data/1(Rst)
  scale_Quality/1 -> NREL UDP Data - Formatted Packets/8("PowerQuality ")
  [TestSeq] -> DMS_Scaling1/1
  DMS_Scaling1/1 -> DMS_Modbus/1
  MGC_controller/1(MGC_controller) -> NREL UDP Data - Formatted Packets/9(MgcCtrl)
  [GOOSE_RX] -> Bus Creator1/9  "GOOSE_RX"

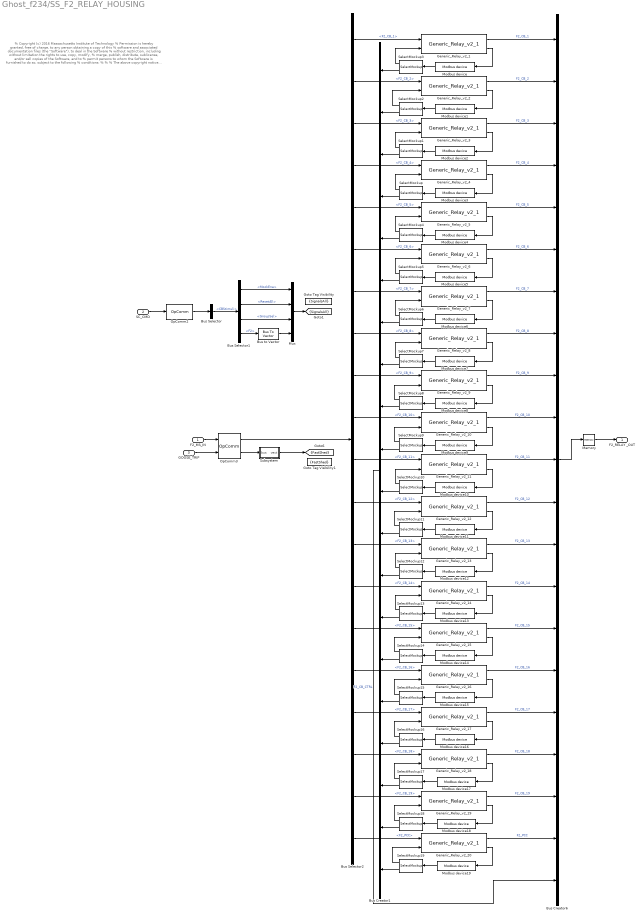
== system Ghost_f234/SS_F2_RELAY_HOUSING ==
  note: % Copyright (c) 2016 Massachusetts Institute of Technology
      | % Permission is hereby granted, free of charge, to any person obtaining a copy of this
      | % software and associated documentation files (the "Software"), to deal in the Software
      | % without restriction, including without limitation the rights to use, copy, modify,
      | % merge, publish, distribute, sublicense, and/or sell copies of the Software, and to
      | % permit persons to whom the Software is furnished to do so, subject to the following
      | % conditions:
      | %
      | %
      | % The above copyright notice and this permission notice shall be included in
      | % all copies or substantial portions of the Software.
      | %
      | % THE SOFTWARE IS PROVIDED "AS IS", WITHOUT WARRANTY OF ANY KIND, EXPRESS OR IMPLIED,
      | % INCLUDING BUT NOT LIMITED TO THE WARRANTIES OF MERCHANTABILITY, FITNESS FOR A
      | % PARTICULAR PURPOSE AND NONINFRINGEMENT. IN NO EVENT SHALL THE AUTHORS OR COPYRIGHT
      | % HOLDERS BE LIABLE FOR ANY CLAIM, DAMAGES OR OTHER LIABILITY, WHETHER IN AN ACTION
      | % OF CONTRACT, TORT OR OTHERWISE, ARISING FROM, OUT OF OR IN CONNECTION WITH THE
      | % SOFTWARE OR THE USE OR OTHER DEALINGS IN THE SOFTWARE.
      | %
      | %
      | %%
  F2_MS_IN : Inport
  SC_CMD : Inport  Port=2
  GOOSE_TRIP : Inport  Port=3
  Bus Creator1 : BusCreator  Inputs=20
  Bus Creator6 : BusCreator  Inputs=21
  Bus Selector : BusSelector  OutputSignals=CBStimuli
  Bus Selector1 : BusSelector  OutputSignals=MockEna,ResetAll,GroupSel,F2
  Bus Selector2 : BusSelector  OutputSignals=CB_DATA.F2_CB_1,CB_DATA.F2_CB_2,CB_DATA.F2_CB_3,CB_DATA.F2_CB_4,CB_DATA.F2_CB_5,CB_DATA.F2_CB_6,CB_DATA.F2_CB_7,CB_DATA.F2_CB_8,CB_DATA.F2_CB_9,CB_DATA.F2_CB_10,CB_DATA.F2_CB_11,CB_DATA.F2_CB_12,CB_DATA.F2_CB_13,CB_DATA.F2_CB_14,CB_DATA.F2_CB_15,CB_DATA.F2_CB_16,CB_DATA.F2_CB_17,CB_DATA.F2_CB_18,CB_DATA.F2_CB_19,CB_DATA.F2_PCC
  Bus to Vector : BusToVector
  Generic_Relay_v2_1 : relay_modbus_lib/Generic_Relay_v2_1  Ts=Ts  relay_settings=[F2(1,:)]
  Generic_Relay_v2_10 : relay_modbus_lib/Generic_Relay_v2_1  Ts=Ts  relay_settings=[F2(10,:)]
  Generic_Relay_v2_11 : relay_modbus_lib/Generic_Relay_v2_1  Ts=Ts  relay_settings=[F2(11,:)]
  Generic_Relay_v2_12 : relay_modbus_lib/Generic_Relay_v2_1  Ts=Ts  relay_settings=[F2(12,:)]
  Generic_Relay_v2_13 : relay_modbus_lib/Generic_Relay_v2_1  Ts=Ts  relay_settings=[F2(13,:)]
  Generic_Relay_v2_14 : relay_modbus_lib/Generic_Relay_v2_1  Ts=Ts  relay_settings=[F2(14,:)]
  Generic_Relay_v2_15 : relay_modbus_lib/Generic_Relay_v2_1  Ts=Ts  relay_settings=[F2(15,:)]
  Generic_Relay_v2_16 : relay_modbus_lib/Generic_Relay_v2_1  Ts=Ts  relay_settings=[F2(16,:)]
  Generic_Relay_v2_17 : relay_modbus_lib/Generic_Relay_v2_1  Ts=Ts  relay_settings=[F2(17,:)]
  Generic_Relay_v2_18 : relay_modbus_lib/Generic_Relay_v2_1  Ts=Ts  relay_settings=[F2(18,:)]
  Generic_Relay_v2_19 : relay_modbus_lib/Generic_Relay_v2_1  Ts=Ts  relay_settings=[F2(19,:)]
  Generic_Relay_v2_2 : relay_modbus_lib/Generic_Relay_v2_1  Ts=Ts  relay_settings=[F2(2,:)]
  Generic_Relay_v2_20 : relay_modbus_lib/Generic_Relay_v2_1  Ts=Ts  relay_settings=[F0(2,:)]
  Generic_Relay_v2_3 : relay_modbus_lib/Generic_Relay_v2_1  Ts=Ts  relay_settings=[F2(3,:)]
  Generic_Relay_v2_4 : relay_modbus_lib/Generic_Relay_v2_1  Ts=Ts  relay_settings=[F2(4,:)]
  Generic_Relay_v2_5 : relay_modbus_lib/Generic_Relay_v2_1  Ts=Ts  relay_settings=[F2(5,:)]
  Generic_Relay_v2_6 : relay_modbus_lib/Generic_Relay_v2_1  Ts=Ts  relay_settings=[F2(6,:)]
  Generic_Relay_v2_7 : relay_modbus_lib/Generic_Relay_v2_1  Ts=Ts  relay_settings=[F2(7,:)]
  Generic_Relay_v2_8 : relay_modbus_lib/Generic_Relay_v2_1  Ts=Ts  relay_settings=[F2(8,:)]
  Generic_Relay_v2_9 : relay_modbus_lib/Generic_Relay_v2_1  Ts=Ts  relay_settings=[F2(9,:)]
  Goto Tag Visibility : GotoTagVisibility  GotoTag=SignalsAll
  Goto Tag Visibility1 : GotoTagVisibility  GotoTag=FastShed
  Memory : Memory
  Modbus device : rtio_generic_modbus/Modbus device  conf_name=F2_relay_cfg1.opal  conf_name_mask=F2_relay_cfg1.xls  sample_time=Ts
  Modbus device1 : rtio_generic_modbus/Modbus device  conf_name=F2_relay_cfg2.opal  conf_name_mask=F2_relay_cfg2.xls  sample_time=Ts
  Modbus device10 : rtio_generic_modbus/Modbus device  conf_name=F2_relay_cfg11.opal  conf_name_mask=F2_relay_cfg11.xls  sample_time=Ts
  Modbus device11 : rtio_generic_modbus/Modbus device  conf_name=F2_relay_cfg12.opal  conf_name_mask=F2_relay_cfg12.xls  sample_time=Ts
  Modbus device12 : rtio_generic_modbus/Modbus device  conf_name=F2_relay_cfg13.opal  conf_name_mask=F2_relay_cfg13.xls  sample_time=Ts
  Modbus device13 : rtio_generic_modbus/Modbus device  conf_name=F2_relay_cfg14.opal  conf_name_mask=F2_relay_cfg14.xls  sample_time=Ts
  Modbus device14 : rtio_generic_modbus/Modbus device  conf_name=F2_relay_cfg15.opal  conf_name_mask=F2_relay_cfg15.xls  sample_time=Ts
  Modbus device15 : rtio_generic_modbus/Modbus device  conf_name=F2_relay_cfg16.opal  conf_name_mask=F2_relay_cfg16.xls  sample_time=Ts
  Modbus device16 : rtio_generic_modbus/Modbus device  conf_name=F2_relay_cfg17.opal  conf_name_mask=F2_relay_cfg17.xls  sample_time=Ts
  Modbus device17 : rtio_generic_modbus/Modbus device  conf_name=F2_relay_cfg18.opal  conf_name_mask=F2_relay_cfg18.xls  sample_time=Ts
  Modbus device18 : rtio_generic_modbus/Modbus device  conf_name=F2_relay_cfg19.opal  conf_name_mask=F2_relay_cfg19.xls  sample_time=Ts
  Modbus device19 : rtio_generic_modbus/Modbus device  conf_name=F2_relay_cfg_pcc.opal  conf_name_mask=F2_relay_cfg_pcc.xls  sample_time=Ts
  Modbus device2 : rtio_generic_modbus/Modbus device  conf_name=F2_relay_cfg3.opal  conf_name_mask=F2_relay_cfg3.xls  sample_time=Ts
  Modbus device3 : rtio_generic_modbus/Modbus device  conf_name=F2_relay_cfg4.opal  conf_name_mask=F2_relay_cfg4.xls  sample_time=Ts
  Modbus device4 : rtio_generic_modbus/Modbus device  conf_name=F2_relay_cfg5.opal  conf_name_mask=F2_relay_cfg5.xls  sample_time=Ts
  Modbus device5 : rtio_generic_modbus/Modbus device  conf_name=F2_relay_cfg6.opal  conf_name_mask=F2_relay_cfg6.xls  sample_time=Ts
  Modbus device6 : rtio_generic_modbus/Modbus device  conf_name=F2_relay_cfg7.opal  conf_name_mask=F2_relay_cfg7.xls  sample_time=Ts
  Modbus device7 : rtio_generic_modbus/Modbus device  conf_name=F2_relay_cfg8.opal  conf_name_mask=F2_relay_cfg8.xls  sample_time=Ts
  Modbus device8 : rtio_generic_modbus/Modbus device  conf_name=F2_relay_cfg9.opal  conf_name_mask=F2_relay_cfg9.xls  sample_time=Ts
  Modbus device9 : rtio_generic_modbus/Modbus device  conf_name=F2_relay_cfg10.opal  conf_name_mask=F2_relay_cfg10.xls  sample_time=Ts
  Mux : Mux
  OpComm2 : rtlab/OpComm  nbport=1  groupe_acq=1  subsys_rate=0  st=0  Synchronization=on  Interpolation=on  Threshold=1.0  Missed_Data=off  Sim_Time=off  Samples=off  dynSigOut=off  from_console=0  warning_done=off  writeOpCommFile=off  Offset=off
  OpComm3 : rtlab/OpComm  nbport=2  groupe_acq=1  subsys_rate=0  st=0  Synchronization=on  Interpolation=on  Threshold=1.0  Missed_Data=off  Sim_Time=off  Samples=off  dynSigOut=off  from_console=0  warning_done=off  writeOpCommFile=off  Offset=off
  SelectMockup : relay_modbus_lib/SelectMockup  sigID=4  sigN=20
  SelectMockup1 : relay_modbus_lib/SelectMockup  sigID=3  sigN=20
  SelectMockup10 : relay_modbus_lib/SelectMockup  sigID=11  sigN=20
  SelectMockup11 : relay_modbus_lib/SelectMockup  sigID=12  sigN=20
  SelectMockup12 : relay_modbus_lib/SelectMockup  sigID=13  sigN=20
  SelectMockup13 : relay_modbus_lib/SelectMockup  sigID=14  sigN=20
  SelectMockup14 : relay_modbus_lib/SelectMockup  sigID=15  sigN=20
  SelectMockup15 : relay_modbus_lib/SelectMockup  sigID=16  sigN=20
  SelectMockup16 : relay_modbus_lib/SelectMockup  sigID=17  sigN=20
  SelectMockup17 : relay_modbus_lib/SelectMockup  sigID=18  sigN=20
  SelectMockup18 : relay_modbus_lib/SelectMockup  sigID=19  sigN=20
  SelectMockup19 : relay_modbus_lib/SelectMockup  sigID=20  sigN=20
  SelectMockup2 : relay_modbus_lib/SelectMockup  sigID=2  sigN=20
  SelectMockup3 : relay_modbus_lib/SelectMockup  sigID=1  sigN=20
  SelectMockup4 : relay_modbus_lib/SelectMockup  sigID=5  sigN=20
  SelectMockup5 : relay_modbus_lib/SelectMockup  sigID=6  sigN=20
  SelectMockup6 : relay_modbus_lib/SelectMockup  sigID=7  sigN=20
  SelectMockup7 : relay_modbus_lib/SelectMockup  sigID=8  sigN=20
  SelectMockup8 : relay_modbus_lib/SelectMockup  sigID=9  sigN=20
  SelectMockup9 : relay_modbus_lib/SelectMockup  sigID=10  sigN=20
  Subsystem : Subsystem
  F2_RELAY _OUT : Outport
  tag scope: FastShed=scoped, SignalsAll=scoped
  wires:
  OpComm3/1 -> Bus Selector2/1
  SelectMockup16/1 -> Generic_Relay_v2_17/2
  Generic_Relay_v2_17/2 -> Modbus device16/1
  SelectMockup15/1 -> Generic_Relay_v2_16/2
  Generic_Relay_v2_16/2 -> Modbus device15/1
  SelectMockup14/1 -> Generic_Relay_v2_15/2
  Generic_Relay_v2_15/2 -> Modbus device14/1
  SelectMockup13/1 -> Generic_Relay_v2_14/2
  Generic_Relay_v2_14/2 -> Modbus device13/1
  Generic_Relay_v2_13/2 -> Modbus device12/1
  SelectMockup12/1 -> Generic_Relay_v2_13/2
  SelectMockup11/1 -> Generic_Relay_v2_12/2
  Generic_Relay_v2_12/2 -> Modbus device11/1
  SelectMockup10/1 -> Generic_Relay_v2_11/2
  Generic_Relay_v2_11/2 -> Modbus device10/1
  SelectMockup9/1 -> Generic_Relay_v2_10/2
  Generic_Relay_v2_10/2 -> Modbus device9/1
  SelectMockup8/1 -> Generic_Relay_v2_9/2
  Generic_Relay_v2_9/2 -> Modbus device8/1
  SelectMockup7/1 -> Generic_Relay_v2_8/2
  Generic_Relay_v2_8/2 -> Modbus device7/1
  SelectMockup6/1 -> Generic_Relay_v2_7/2
  Generic_Relay_v2_7/2 -> Modbus device6/1
  Generic_Relay_v2_6/2 -> Modbus device5/1
  SelectMockup5/1 -> Generic_Relay_v2_6/2
  SelectMockup4/1 -> Generic_Relay_v2_5/2
  Generic_Relay_v2_5/2 -> Modbus device4/1
  SelectMockup/1 -> Generic_Relay_v2_4/2
  Generic_Relay_v2_4/2 -> Modbus device3/1
  SelectMockup1/1 -> Generic_Relay_v2_3/2
  Generic_Relay_v2_3/2 -> Modbus device2/1
  SelectMockup2/1 -> Generic_Relay_v2_2/2
  Generic_Relay_v2_2/2 -> Modbus device1/1
  SelectMockup3/1 -> Generic_Relay_v2_1/2
  Generic_Relay_v2_1/2 -> Modbus device/1
  Bus Creator6/1 -> Memory/1
  F2_MS_IN/1 -> OpComm3/1
  Bus Selector2/1 -> Generic_Relay_v2_1/1  "<F2_CB_1>"
  Generic_Relay_v2_1/1 -> Bus Creator6/1  "F2_CB_1"
  Bus Selector2/2 -> Generic_Relay_v2_2/1  "<F2_CB_2>"
  Bus Selector2/3 -> Generic_Relay_v2_3/1  "<F2_CB_3>"
  Bus Selector2/4 -> Generic_Relay_v2_4/1  "<F2_CB_4>"
  Bus Selector2/5 -> Generic_Relay_v2_5/1  "<F2_CB_5>"
  Bus Selector2/6 -> Generic_Relay_v2_6/1  "<F2_CB_6>"
  Bus Selector2/7 -> Generic_Relay_v2_7/1  "<F2_CB_7>"
  Bus Selector2/8 -> Generic_Relay_v2_8/1  "<F2_CB_8>"
  Bus Selector2/9 -> Generic_Relay_v2_9/1  "<F2_CB_9>"
  Bus Selector2/10 -> Generic_Relay_v2_10/1  "<F2_CB_10>"
  Bus Selector2/11 -> Generic_Relay_v2_11/1  "<F2_CB_11>"
  Bus Selector2/12 -> Generic_Relay_v2_12/1  "<F2_CB_12>"
  Bus Selector2/13 -> Generic_Relay_v2_13/1  "<F2_CB_13>"
  Bus Selector2/14 -> Generic_Relay_v2_14/1  "<F2_CB_14>"
  Bus Selector2/15 -> Generic_Relay_v2_15/1  "<F2_CB_15>"
  Bus Selector2/16 -> Generic_Relay_v2_16/1  "<F2_CB_16>"
  Generic_Relay_v2_12/1 -> Bus Creator6/12  "F2_CB_12"
  Generic_Relay_v2_13/1 -> Bus Creator6/13  "F2_CB_13"
  Generic_Relay_v2_14/1 -> Bus Creator6/14  "F2_CB_14"
  Generic_Relay_v2_15/1 -> Bus Creator6/15  "F2_CB_15"
  Generic_Relay_v2_16/1 -> Bus Creator6/16  "F2_CB_16"
  Generic_Relay_v2_11/1 -> Bus Creator6/11  "F2_CB_11"
  Generic_Relay_v2_10/1 -> Bus Creator6/10  "F2_CB_10"
  Generic_Relay_v2_9/1 -> Bus Creator6/9  "F2_CB_9"
  Generic_Relay_v2_8/1 -> Bus Creator6/8  "F2_CB_8"
  Generic_Relay_v2_7/1 -> Bus Creator6/7  "F2_CB_7"
  Generic_Relay_v2_2/1 -> Bus Creator6/2  "F2_CB_2"
  Generic_Relay_v2_3/1 -> Bus Creator6/3  "F2_CB_3"
  Generic_Relay_v2_4/1 -> Bus Creator6/4  "F2_CB_4"
  Generic_Relay_v2_5/1 -> Bus Creator6/5  "F2_CB_5"
  Generic_Relay_v2_6/1 -> Bus Creator6/6  "F2_CB_6"
  Generic_Relay_v2_17/1 -> Bus Creator6/17  "F2_CB_17"
  Bus Selector2/17 -> Generic_Relay_v2_17/1  "<F2_CB_17>"
  SelectMockup18/1 -> Generic_Relay_v2_19/2
  Generic_Relay_v2_19/2 -> Modbus device18/1
  SelectMockup17/1 -> Generic_Relay_v2_18/2
  Generic_Relay_v2_18/2 -> Modbus device17/1
  Generic_Relay_v2_18/1 -> Bus Creator6/18  "F2_CB_18"
  Generic_Relay_v2_19/1 -> Bus Creator6/19  "F2_CB_19"
  Bus Selector2/19 -> Generic_Relay_v2_19/1  "<F2_CB_19>"
  Bus Selector2/18 -> Generic_Relay_v2_18/1  "<F2_CB_18>"
  Memory/1 -> F2_RELAY _OUT/1
  SelectMockup19/1 -> Generic_Relay_v2_20/2
  Generic_Relay_v2_20/2 -> Modbus device19/1
  Generic_Relay_v2_20/1 -> Bus Creator6/20  "F2_PCC"
  Bus Selector2/20 -> Generic_Relay_v2_20/1  "<F2_PCC>"
  Modbus device18/1 -> SelectMockup18/1
  Modbus device17/1 -> SelectMockup17/1
  Modbus device16/1 -> SelectMockup16/1
  Modbus device15/1 -> SelectMockup15/1
  Modbus device14/1 -> SelectMockup14/1
  Modbus device13/1 -> SelectMockup13/1
  Modbus device12/1 -> SelectMockup12/1
  Modbus device11/1 -> SelectMockup11/1
  Modbus device10/1 -> SelectMockup10/1
  Modbus device9/1 -> SelectMockup9/1
  Modbus device8/1 -> SelectMockup8/1
  Modbus device7/1 -> SelectMockup7/1
  Modbus device6/1 -> SelectMockup6/1
  Modbus device5/1 -> SelectMockup5/1
  Modbus device4/1 -> SelectMockup4/1
  Modbus device3/1 -> SelectMockup/1
  Modbus device2/1 -> SelectMockup1/1
  Modbus device1/1 -> SelectMockup2/1
  Modbus device/1 -> SelectMockup3/1
  Modbus device19/1 -> SelectMockup19/1
  SC_CMD/1 -> OpComm2/1
  OpComm2/1 -> Bus Selector/1
  Bus Selector/1 -> Bus Selector1/1  "<CBStimuli>"
  Bus Selector1/4 -> Bus to Vector/1  "<F2>"
  Bus Selector1/1 -> Mux/1  "<MockEna>"
  Bus to Vector/1 -> Mux/4
  Bus Selector1/3 -> Mux/3  "<GroupSel>"
  Bus Selector1/2 -> Mux/2  "<ResetAll>"
  Mux/1 -> [SignalsAll]
  GOOSE_TRIP/1 -> OpComm3/2
  OpComm3/2 -> Subsystem/1(bus)
  Subsystem/1(vect) -> [FastShed]
  SelectMockup3/2 -> Bus Creator1/1
  SelectMockup2/2 -> Bus Creator1/2
  SelectMockup1/2 -> Bus Creator1/3
  SelectMockup/2 -> Bus Creator1/4
  SelectMockup4/2 -> Bus Creator1/5
  SelectMockup5/2 -> Bus Creator1/6
  SelectMockup6/2 -> Bus Creator1/7
  SelectMockup7/2 -> Bus Creator1/8
  SelectMockup8/2 -> Bus Creator1/9
  SelectMockup9/2 -> Bus Creator1/10
  Bus Creator1/1 -> Bus Creator6/21  "F2_CB_CTRL"
  SelectMockup10/2 -> Bus Creator1/11
  SelectMockup11/2 -> Bus Creator1/12
  SelectMockup12/2 -> Bus Creator1/13
  SelectMockup13/2 -> Bus Creator1/14
  SelectMockup14/2 -> Bus Creator1/15
  SelectMockup15/2 -> Bus Creator1/16
  SelectMockup16/2 -> Bus Creator1/17
  SelectMockup17/2 -> Bus Creator1/18
  SelectMockup18/2 -> Bus Creator1/19
  SelectMockup19/2 -> Bus Creator1/20
